simulink library "BEML_EMU_DoorsInput_Lib"  (R2019b)
settings: Solver=VariableStepAuto  StartTime=0.0  StopTime=10.0  RelTol=1e-3
undefined symbols (not defined in the file): DoorsSampleTime, DoorWinder, ElectricalSignals, EmerDoorLatched, EmerDoorOpenFault, EmergencyDoorGasSpring, EmergencyDoorHandle, EmergencyDoorMechanicalUnlocked, HasCab, InputControlStates, RampCoverLockingLever, RampHandle, RampMiddleSupport, RampWinder
libraries: simulink x128, $bdroot x8, VectorOperationsLib x1
(part 2 of 2)

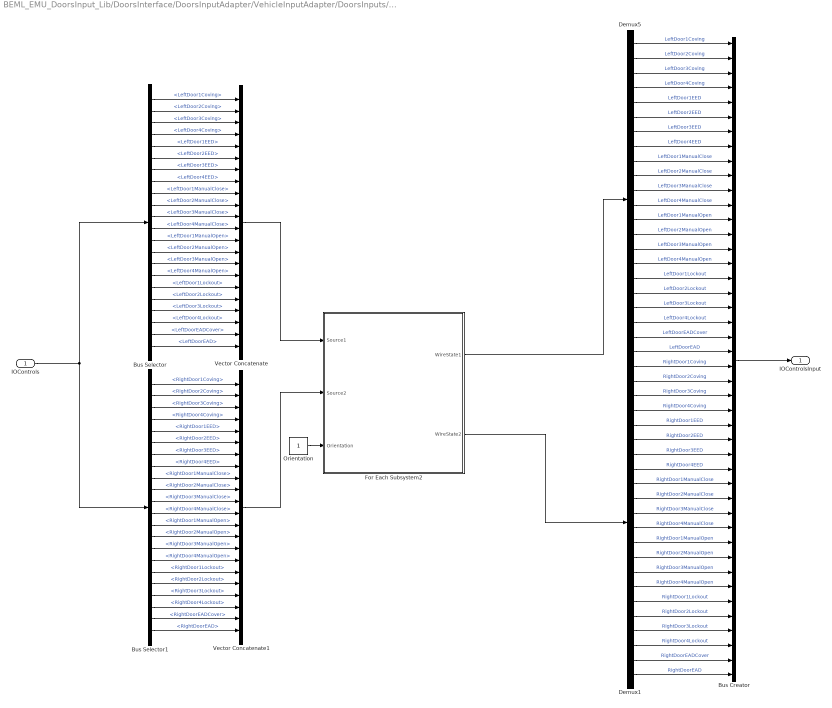
== system BEML_EMU_DoorsInput_Lib/DoorsInterface/DoorsInputAdapter/VehicleInputAdapter/DoorsInputs/DoorsArrangement/Subsystem1 ==
  IOControls : Inport
  Bus Creator : BusCreator  Inputs=LeftDoor1Coving,LeftDoor2Coving,LeftDoor3Coving,LeftDoor4Coving,LeftDoor1EED,LeftDoor2EED,LeftDoor3EED,LeftDoor4EED,LeftDoor1ManualClose,LeftDoor2ManualClose,LeftDoor3ManualClose,LeftDoor4ManualClose,LeftDoor1ManualOpen,LeftDoor2ManualOpen,LeftDoor3ManualOpen,LeftDoor4ManualOpen,LeftDoor1Lockout,LeftDoor2Lockout,LeftDoor3Lockout,LeftDoor4Lockout,LeftDoorEADCover,LeftDoorEAD,RightDoor1Coving,RightDoor2Coving,RightDoor3Coving,RightDoor4Coving,RightDoor1EED,RightDoor2EED,RightDoor3EED,RightDoor4EED,RightDoor1ManualClose,RightDoor2ManualClose,RightDoor3ManualClose,RightDoor4ManualClose,RightDoor1ManualOpen,RightDoor2ManualOpen,RightDoor3ManualOpen,RightDoor4ManualOpen,RightDoor1Lockout,RightDoor2Lockout,RightDoor3Lockout,RightDoor4Lockout,RightDoorEADCover,RightDoorEAD
  Bus Selector : BusSelector  OutputSignals=LeftDoor1Coving,LeftDoor2Coving,LeftDoor3Coving,LeftDoor4Coving,LeftDoor1EED,LeftDoor2EED,LeftDoor3EED,LeftDoor4EED,LeftDoor1ManualClose,LeftDoor2ManualClose,LeftDoor3ManualClose,LeftDoor4ManualClose,LeftDoor1ManualOpen,LeftDoor2ManualOpen,LeftDoor3ManualOpen,LeftDoor4ManualOpen,LeftDoor1Lockout,LeftDoor2Lockout,LeftDoor3Lockout,LeftDoor4Lockout,LeftDoorEADCover,LeftDoorEAD
  Bus Selector1 : BusSelector  OutputSignals=RightDoor1Coving,RightDoor2Coving,RightDoor3Coving,RightDoor4Coving,RightDoor1EED,RightDoor2EED,RightDoor3EED,RightDoor4EED,RightDoor1ManualClose,RightDoor2ManualClose,RightDoor3ManualClose,RightDoor4ManualClose,RightDoor1ManualOpen,RightDoor2ManualOpen,RightDoor3ManualOpen,RightDoor4ManualOpen,RightDoor1Lockout,RightDoor2Lockout,RightDoor3Lockout,RightDoor4Lockout,RightDoorEADCover,RightDoorEAD
  Demux1 : Demux  Outputs=22
  Demux5 : Demux  Outputs=22
  For Each Subsystem2 : Subsystem  TreatAsAtomicUnit=on
  Orientation : Constant
  Vector Concatenate : Concatenate  NumInputs=22
  Vector Concatenate1 : Concatenate  NumInputs=22
  IOControlsInput : Outport
  wires:
  Bus Selector/22 -> Vector Concatenate/22  "<LeftDoorEAD>"
  Bus Selector/21 -> Vector Concatenate/21  "<LeftDoorEADCover>"
  Bus Selector/1 -> Vector Concatenate/1  "<LeftDoor1Coving>"
  Bus Selector/2 -> Vector Concatenate/2  "<LeftDoor2Coving>"
  Bus Selector/3 -> Vector Concatenate/3  "<LeftDoor3Coving>"
  Bus Selector/4 -> Vector Concatenate/4  "<LeftDoor4Coving>"
  Bus Selector/5 -> Vector Concatenate/5  "<LeftDoor1EED>"
  Bus Selector/6 -> Vector Concatenate/6  "<LeftDoor2EED>"
  Bus Selector/7 -> Vector Concatenate/7  "<LeftDoor3EED>"
  Bus Selector/8 -> Vector Concatenate/8  "<LeftDoor4EED>"
  Bus Selector/9 -> Vector Concatenate/9  "<LeftDoor1ManualClose>"
  Bus Selector/10 -> Vector Concatenate/10  "<LeftDoor2ManualClose>"
  Bus Selector/11 -> Vector Concatenate/11  "<LeftDoor3ManualClose>"
  Bus Selector/12 -> Vector Concatenate/12  "<LeftDoor4ManualClose>"
  Bus Selector/13 -> Vector Concatenate/13  "<LeftDoor1ManualOpen>"
  Bus Selector/14 -> Vector Concatenate/14  "<LeftDoor2ManualOpen>"
  Bus Selector/15 -> Vector Concatenate/15  "<LeftDoor3ManualOpen>"
  Bus Selector/16 -> Vector Concatenate/16  "<LeftDoor4ManualOpen>"
  Bus Selector/17 -> Vector Concatenate/17  "<LeftDoor1Lockout>"
  Bus Selector/18 -> Vector Concatenate/18  "<LeftDoor2Lockout>"
  Bus Selector/19 -> Vector Concatenate/19  "<LeftDoor3Lockout>"
  Bus Selector/20 -> Vector Concatenate/20  "<LeftDoor4Lockout>"
  Bus Selector1/20 -> Vector Concatenate1/20  "<RightDoor4Lockout>"
  Bus Selector1/19 -> Vector Concatenate1/19  "<RightDoor3Lockout>"
  Bus Selector1/18 -> Vector Concatenate1/18  "<RightDoor2Lockout>"
  Bus Selector1/17 -> Vector Concatenate1/17  "<RightDoor1Lockout>"
  Bus Selector1/16 -> Vector Concatenate1/16  "<RightDoor4ManualOpen>"
  Bus Selector1/15 -> Vector Concatenate1/15  "<RightDoor3ManualOpen>"
  Bus Selector1/14 -> Vector Concatenate1/14  "<RightDoor2ManualOpen>"
  Bus Selector1/13 -> Vector Concatenate1/13  "<RightDoor1ManualOpen>"
  Bus Selector1/12 -> Vector Concatenate1/12  "<RightDoor4ManualClose>"
  Bus Selector1/11 -> Vector Concatenate1/11  "<RightDoor3ManualClose>"
  Bus Selector1/10 -> Vector Concatenate1/10  "<RightDoor2ManualClose>"
  Bus Selector1/9 -> Vector Concatenate1/9  "<RightDoor1ManualClose>"
  Bus Selector1/8 -> Vector Concatenate1/8  "<RightDoor4EED>"
  Bus Selector1/7 -> Vector Concatenate1/7  "<RightDoor3EED>"
  Bus Selector1/6 -> Vector Concatenate1/6  "<RightDoor2EED>"
  Bus Selector1/5 -> Vector Concatenate1/5  "<RightDoor1EED>"
  Bus Selector1/4 -> Vector Concatenate1/4  "<RightDoor4Coving>"
  Bus Selector1/3 -> Vector Concatenate1/3  "<RightDoor3Coving>"
  Bus Selector1/2 -> Vector Concatenate1/2  "<RightDoor2Coving>"
  Bus Selector1/1 -> Vector Concatenate1/1  "<RightDoor1Coving>"
  Bus Selector1/21 -> Vector Concatenate1/21  "<RightDoorEADCover>"
  Bus Selector1/22 -> Vector Concatenate1/22  "<RightDoorEAD>"
  IOControls/1 -> Bus Selector/1, Bus Selector1/1
  Vector Concatenate/1 -> For Each Subsystem2/1(Source1)
  Vector Concatenate1/1 -> For Each Subsystem2/2(Source2)
  For Each Subsystem2/2(WireState2) -> Demux1/1
  For Each Subsystem2/1(WireState1) -> Demux5/1
  Demux5/22 -> Bus Creator/22  "LeftDoorEAD"
  Demux5/21 -> Bus Creator/21  "LeftDoorEADCover"
  Demux5/20 -> Bus Creator/20  "LeftDoor4Lockout"
  Demux5/19 -> Bus Creator/19  "LeftDoor3Lockout"
  Demux5/18 -> Bus Creator/18  "LeftDoor2Lockout"
  Demux5/17 -> Bus Creator/17  "LeftDoor1Lockout"
  Demux5/16 -> Bus Creator/16  "LeftDoor4ManualOpen"
  Demux5/15 -> Bus Creator/15  "LeftDoor3ManualOpen"
  Demux5/14 -> Bus Creator/14  "LeftDoor2ManualOpen"
  Demux5/13 -> Bus Creator/13  "LeftDoor1ManualOpen"
  Demux5/12 -> Bus Creator/12  "LeftDoor4ManualClose"
  Demux5/11 -> Bus Creator/11  "LeftDoor3ManualClose"
  Demux5/10 -> Bus Creator/10  "LeftDoor2ManualClose"
  Demux5/9 -> Bus Creator/9  "LeftDoor1ManualClose"
  Demux5/8 -> Bus Creator/8  "LeftDoor4EED"
  Demux5/7 -> Bus Creator/7  "LeftDoor3EED"
  Demux5/6 -> Bus Creator/6  "LeftDoor2EED"
  Demux5/5 -> Bus Creator/5  "LeftDoor1EED"
  Demux5/4 -> Bus Creator/4  "LeftDoor4Coving"
  Demux5/3 -> Bus Creator/3  "LeftDoor3Coving"
  Demux5/2 -> Bus Creator/2  "LeftDoor2Coving"
  Demux5/1 -> Bus Creator/1  "LeftDoor1Coving"
  Demux1/1 -> Bus Creator/23  "RightDoor1Coving"
  Demux1/2 -> Bus Creator/24  "RightDoor2Coving"
  Demux1/3 -> Bus Creator/25  "RightDoor3Coving"
  Demux1/4 -> Bus Creator/26  "RightDoor4Coving"
  Demux1/5 -> Bus Creator/27  "RightDoor1EED"
  Demux1/6 -> Bus Creator/28  "RightDoor2EED"
  Demux1/7 -> Bus Creator/29  "RightDoor3EED"
  Demux1/8 -> Bus Creator/30  "RightDoor4EED"
  Demux1/9 -> Bus Creator/31  "RightDoor1ManualClose"
  Demux1/10 -> Bus Creator/32  "RightDoor2ManualClose"
  Demux1/11 -> Bus Creator/33  "RightDoor3ManualClose"
  Demux1/12 -> Bus Creator/34  "RightDoor4ManualClose"
  Demux1/13 -> Bus Creator/35  "RightDoor1ManualOpen"
  Demux1/14 -> Bus Creator/36  "RightDoor2ManualOpen"
  Demux1/15 -> Bus Creator/37  "RightDoor3ManualOpen"
  Demux1/16 -> Bus Creator/38  "RightDoor4ManualOpen"
  Demux1/17 -> Bus Creator/39  "RightDoor1Lockout"
  Demux1/18 -> Bus Creator/40  "RightDoor2Lockout"
  Demux1/19 -> Bus Creator/41  "RightDoor3Lockout"
  Demux1/20 -> Bus Creator/42  "RightDoor4Lockout"
  Demux1/21 -> Bus Creator/43  "RightDoorEADCover"
  Demux1/22 -> Bus Creator/44  "RightDoorEAD"
  Bus Creator/1 -> IOControlsInput/1
  Orientation/1 -> For Each Subsystem2/3(Orientation)

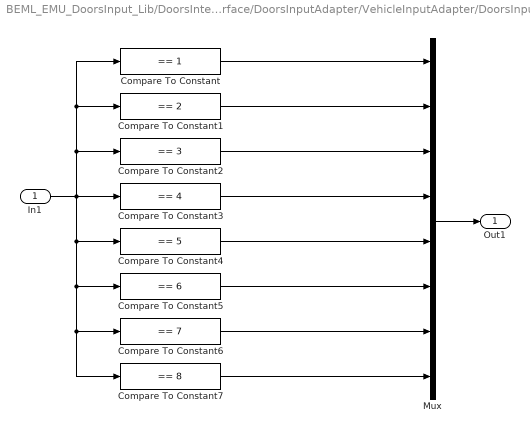
== system BEML_EMU_DoorsInput_Lib/DoorsInterface/DoorsInputAdapter/VehicleInputAdapter/DoorsInputs/Subsystem/Subsystem ==
  In1 : Inport
  Compare To Constant : simulink/Logic and Bit Operations/Compare To Constant  relop===  const=1  OutDataTypeStr=boolean
  Compare To Constant1 : simulink/Logic and Bit Operations/Compare To Constant  relop===  const=2  OutDataTypeStr=boolean
  Compare To Constant2 : simulink/Logic and Bit Operations/Compare To Constant  relop===  const=3  OutDataTypeStr=boolean
  Compare To Constant3 : simulink/Logic and Bit Operations/Compare To Constant  relop===  const=4  OutDataTypeStr=boolean
  Compare To Constant4 : simulink/Logic and Bit Operations/Compare To Constant  relop===  const=5  OutDataTypeStr=boolean
  Compare To Constant5 : simulink/Logic and Bit Operations/Compare To Constant  relop===  const=6  OutDataTypeStr=boolean
  Compare To Constant6 : simulink/Logic and Bit Operations/Compare To Constant  relop===  const=7  OutDataTypeStr=boolean
  Compare To Constant7 : simulink/Logic and Bit Operations/Compare To Constant  relop===  const=8  OutDataTypeStr=boolean
  Mux : Mux  Inputs=8
  Out1 : Outport
  wires:
  Compare To Constant7/1 -> Mux/8
  Compare To Constant6/1 -> Mux/7
  Compare To Constant5/1 -> Mux/6
  Compare To Constant4/1 -> Mux/5
  Compare To Constant3/1 -> Mux/4
  Compare To Constant2/1 -> Mux/3
  Compare To Constant1/1 -> Mux/2
  Compare To Constant/1 -> Mux/1
  Mux/1 -> Out1/1
  In1/1 -> Compare To Constant4/1, Compare To Constant5/1, Compare To Constant6/1, Compare To Constant7/1, Compare To Constant3/1, Compare To Constant2/1, Compare To Constant1/1, Compare To Constant/1

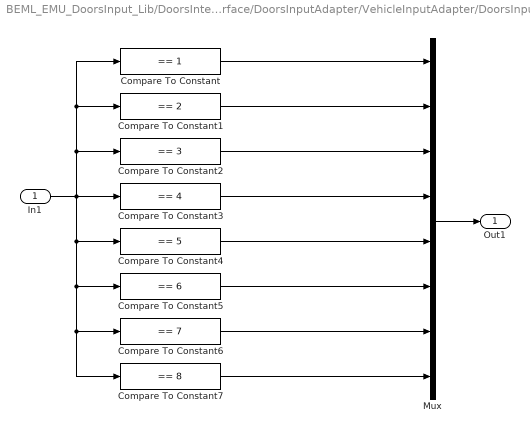
== system BEML_EMU_DoorsInput_Lib/DoorsInterface/DoorsInputAdapter/VehicleInputAdapter/DoorsInputs/Subsystem/Subsystem1 ==
  In1 : Inport
  Compare To Constant : simulink/Logic and Bit Operations/Compare To Constant  relop===  const=1  OutDataTypeStr=boolean
  Compare To Constant1 : simulink/Logic and Bit Operations/Compare To Constant  relop===  const=2  OutDataTypeStr=boolean
  Compare To Constant2 : simulink/Logic and Bit Operations/Compare To Constant  relop===  const=3  OutDataTypeStr=boolean
  Compare To Constant3 : simulink/Logic and Bit Operations/Compare To Constant  relop===  const=4  OutDataTypeStr=boolean
  Compare To Constant4 : simulink/Logic and Bit Operations/Compare To Constant  relop===  const=5  OutDataTypeStr=boolean
  Compare To Constant5 : simulink/Logic and Bit Operations/Compare To Constant  relop===  const=6  OutDataTypeStr=boolean
  Compare To Constant6 : simulink/Logic and Bit Operations/Compare To Constant  relop===  const=7  OutDataTypeStr=boolean
  Compare To Constant7 : simulink/Logic and Bit Operations/Compare To Constant  relop===  const=8  OutDataTypeStr=boolean
  Mux : Mux  Inputs=8
  Out1 : Outport
  wires:
  In1/1 -> Compare To Constant/1, Compare To Constant1/1, Compare To Constant2/1, Compare To Constant3/1, Compare To Constant7/1, Compare To Constant6/1, Compare To Constant5/1, Compare To Constant4/1
  Mux/1 -> Out1/1
  Compare To Constant/1 -> Mux/1
  Compare To Constant1/1 -> Mux/2
  Compare To Constant2/1 -> Mux/3
  Compare To Constant3/1 -> Mux/4
  Compare To Constant4/1 -> Mux/5
  Compare To Constant5/1 -> Mux/6
  Compare To Constant6/1 -> Mux/7
  Compare To Constant7/1 -> Mux/8

== system BEML_EMU_DoorsInput_Lib/DoorsInterface/DoorsInputAdapter/VehicleInputAdapter/DoorsInputs/Subsystem/Subsystem10 ==
  In1 : Inport
  Compare To Constant : simulink/Logic and Bit Operations/Compare To Constant  relop===  const=1  OutDataTypeStr=boolean
  Compare To Constant1 : simulink/Logic and Bit Operations/Compare To Constant  relop===  const=2  OutDataTypeStr=boolean
  Compare To Constant2 : simulink/Logic and Bit Operations/Compare To Constant  relop===  const=3  OutDataTypeStr=boolean
  Compare To Constant3 : simulink/Logic and Bit Operations/Compare To Constant  relop===  const=4  OutDataTypeStr=boolean
  Compare To Constant4 : simulink/Logic and Bit Operations/Compare To Constant  relop===  const=5  OutDataTypeStr=boolean
  Compare To Constant5 : simulink/Logic and Bit Operations/Compare To Constant  relop===  const=6  OutDataTypeStr=boolean
  Compare To Constant6 : simulink/Logic and Bit Operations/Compare To Constant  relop===  const=7  OutDataTypeStr=boolean
  Compare To Constant7 : simulink/Logic and Bit Operations/Compare To Constant  relop===  const=8  OutDataTypeStr=boolean
  Mux : Mux  Inputs=8
  Out1 : Outport
  wires:
  Compare To Constant7/1 -> Mux/8
  Compare To Constant6/1 -> Mux/7
  Compare To Constant5/1 -> Mux/6
  Compare To Constant4/1 -> Mux/5
  Compare To Constant3/1 -> Mux/4
  Compare To Constant2/1 -> Mux/3
  Compare To Constant1/1 -> Mux/2
  Compare To Constant/1 -> Mux/1
  Mux/1 -> Out1/1
  In1/1 -> Compare To Constant4/1, Compare To Constant5/1, Compare To Constant6/1, Compare To Constant7/1, Compare To Constant3/1, Compare To Constant2/1, Compare To Constant1/1, Compare To Constant/1

== system BEML_EMU_DoorsInput_Lib/DoorsInterface/DoorsInputAdapter/VehicleInputAdapter/DoorsInputs/Subsystem/Subsystem11 ==
  In1 : Inport
  Compare To Constant : simulink/Logic and Bit Operations/Compare To Constant  relop===  const=1  OutDataTypeStr=boolean
  Compare To Constant1 : simulink/Logic and Bit Operations/Compare To Constant  relop===  const=2  OutDataTypeStr=boolean
  Compare To Constant2 : simulink/Logic and Bit Operations/Compare To Constant  relop===  const=3  OutDataTypeStr=boolean
  Compare To Constant3 : simulink/Logic and Bit Operations/Compare To Constant  relop===  const=4  OutDataTypeStr=boolean
  Compare To Constant4 : simulink/Logic and Bit Operations/Compare To Constant  relop===  const=5  OutDataTypeStr=boolean
  Compare To Constant5 : simulink/Logic and Bit Operations/Compare To Constant  relop===  const=6  OutDataTypeStr=boolean
  Compare To Constant6 : simulink/Logic and Bit Operations/Compare To Constant  relop===  const=7  OutDataTypeStr=boolean
  Compare To Constant7 : simulink/Logic and Bit Operations/Compare To Constant  relop===  const=8  OutDataTypeStr=boolean
  Mux : Mux  Inputs=8
  Out1 : Outport
  wires:
  In1/1 -> Compare To Constant/1, Compare To Constant1/1, Compare To Constant2/1, Compare To Constant3/1, Compare To Constant7/1, Compare To Constant6/1, Compare To Constant5/1, Compare To Constant4/1
  Mux/1 -> Out1/1
  Compare To Constant/1 -> Mux/1
  Compare To Constant1/1 -> Mux/2
  Compare To Constant2/1 -> Mux/3
  Compare To Constant3/1 -> Mux/4
  Compare To Constant4/1 -> Mux/5
  Compare To Constant5/1 -> Mux/6
  Compare To Constant6/1 -> Mux/7
  Compare To Constant7/1 -> Mux/8

== system BEML_EMU_DoorsInput_Lib/DoorsInterface/DoorsInputAdapter/VehicleInputAdapter/DoorsInputs/Subsystem/Subsystem12 ==
  In1 : Inport
  Compare To Constant : simulink/Logic and Bit Operations/Compare To Constant  relop===  const=1  OutDataTypeStr=boolean
  Compare To Constant1 : simulink/Logic and Bit Operations/Compare To Constant  relop===  const=2  OutDataTypeStr=boolean
  Compare To Constant2 : simulink/Logic and Bit Operations/Compare To Constant  relop===  const=3  OutDataTypeStr=boolean
  Compare To Constant3 : simulink/Logic and Bit Operations/Compare To Constant  relop===  const=4  OutDataTypeStr=boolean
  Compare To Constant4 : simulink/Logic and Bit Operations/Compare To Constant  relop===  const=5  OutDataTypeStr=boolean
  Compare To Constant5 : simulink/Logic and Bit Operations/Compare To Constant  relop===  const=6  OutDataTypeStr=boolean
  Compare To Constant6 : simulink/Logic and Bit Operations/Compare To Constant  relop===  const=7  OutDataTypeStr=boolean
  Compare To Constant7 : simulink/Logic and Bit Operations/Compare To Constant  relop===  const=8  OutDataTypeStr=boolean
  Mux : Mux  Inputs=8
  Out1 : Outport
  wires:
  Compare To Constant7/1 -> Mux/8
  Compare To Constant6/1 -> Mux/7
  Compare To Constant5/1 -> Mux/6
  Compare To Constant4/1 -> Mux/5
  Compare To Constant3/1 -> Mux/4
  Compare To Constant2/1 -> Mux/3
  Compare To Constant1/1 -> Mux/2
  Compare To Constant/1 -> Mux/1
  Mux/1 -> Out1/1
  In1/1 -> Compare To Constant4/1, Compare To Constant5/1, Compare To Constant6/1, Compare To Constant7/1, Compare To Constant3/1, Compare To Constant2/1, Compare To Constant1/1, Compare To Constant/1

== system BEML_EMU_DoorsInput_Lib/DoorsInterface/DoorsInputAdapter/VehicleInputAdapter/DoorsInputs/Subsystem/Subsystem13 ==
  In1 : Inport
  Compare To Constant : simulink/Logic and Bit Operations/Compare To Constant  relop===  const=1  OutDataTypeStr=boolean
  Compare To Constant1 : simulink/Logic and Bit Operations/Compare To Constant  relop===  const=2  OutDataTypeStr=boolean
  Compare To Constant2 : simulink/Logic and Bit Operations/Compare To Constant  relop===  const=3  OutDataTypeStr=boolean
  Compare To Constant3 : simulink/Logic and Bit Operations/Compare To Constant  relop===  const=4  OutDataTypeStr=boolean
  Compare To Constant4 : simulink/Logic and Bit Operations/Compare To Constant  relop===  const=5  OutDataTypeStr=boolean
  Compare To Constant5 : simulink/Logic and Bit Operations/Compare To Constant  relop===  const=6  OutDataTypeStr=boolean
  Compare To Constant6 : simulink/Logic and Bit Operations/Compare To Constant  relop===  const=7  OutDataTypeStr=boolean
  Compare To Constant7 : simulink/Logic and Bit Operations/Compare To Constant  relop===  const=8  OutDataTypeStr=boolean
  Mux : Mux  Inputs=8
  Out1 : Outport
  wires:
  In1/1 -> Compare To Constant/1, Compare To Constant1/1, Compare To Constant2/1, Compare To Constant3/1, Compare To Constant7/1, Compare To Constant6/1, Compare To Constant5/1, Compare To Constant4/1
  Mux/1 -> Out1/1
  Compare To Constant/1 -> Mux/1
  Compare To Constant1/1 -> Mux/2
  Compare To Constant2/1 -> Mux/3
  Compare To Constant3/1 -> Mux/4
  Compare To Constant4/1 -> Mux/5
  Compare To Constant5/1 -> Mux/6
  Compare To Constant6/1 -> Mux/7
  Compare To Constant7/1 -> Mux/8

== system BEML_EMU_DoorsInput_Lib/DoorsInterface/DoorsInputAdapter/VehicleInputAdapter/DoorsInputs/Subsystem/Subsystem14 ==
  In1 : Inport
  Compare To Constant : simulink/Logic and Bit Operations/Compare To Constant  relop===  const=1  OutDataTypeStr=boolean
  Compare To Constant1 : simulink/Logic and Bit Operations/Compare To Constant  relop===  const=2  OutDataTypeStr=boolean
  Compare To Constant2 : simulink/Logic and Bit Operations/Compare To Constant  relop===  const=3  OutDataTypeStr=boolean
  Compare To Constant3 : simulink/Logic and Bit Operations/Compare To Constant  relop===  const=4  OutDataTypeStr=boolean
  Compare To Constant4 : simulink/Logic and Bit Operations/Compare To Constant  relop===  const=5  OutDataTypeStr=boolean
  Compare To Constant5 : simulink/Logic and Bit Operations/Compare To Constant  relop===  const=6  OutDataTypeStr=boolean
  Compare To Constant6 : simulink/Logic and Bit Operations/Compare To Constant  relop===  const=7  OutDataTypeStr=boolean
  Compare To Constant7 : simulink/Logic and Bit Operations/Compare To Constant  relop===  const=8  OutDataTypeStr=boolean
  Mux : Mux  Inputs=8
  Out1 : Outport
  wires:
  Compare To Constant7/1 -> Mux/8
  Compare To Constant6/1 -> Mux/7
  Compare To Constant5/1 -> Mux/6
  Compare To Constant4/1 -> Mux/5
  Compare To Constant3/1 -> Mux/4
  Compare To Constant2/1 -> Mux/3
  Compare To Constant1/1 -> Mux/2
  Compare To Constant/1 -> Mux/1
  Mux/1 -> Out1/1
  In1/1 -> Compare To Constant4/1, Compare To Constant5/1, Compare To Constant6/1, Compare To Constant7/1, Compare To Constant3/1, Compare To Constant2/1, Compare To Constant1/1, Compare To Constant/1

== system BEML_EMU_DoorsInput_Lib/DoorsInterface/DoorsInputAdapter/VehicleInputAdapter/DoorsInputs/Subsystem/Subsystem15 ==
  In1 : Inport
  Compare To Constant : simulink/Logic and Bit Operations/Compare To Constant  relop===  const=1  OutDataTypeStr=boolean
  Compare To Constant1 : simulink/Logic and Bit Operations/Compare To Constant  relop===  const=2  OutDataTypeStr=boolean
  Compare To Constant2 : simulink/Logic and Bit Operations/Compare To Constant  relop===  const=3  OutDataTypeStr=boolean
  Compare To Constant3 : simulink/Logic and Bit Operations/Compare To Constant  relop===  const=4  OutDataTypeStr=boolean
  Compare To Constant4 : simulink/Logic and Bit Operations/Compare To Constant  relop===  const=5  OutDataTypeStr=boolean
  Compare To Constant5 : simulink/Logic and Bit Operations/Compare To Constant  relop===  const=6  OutDataTypeStr=boolean
  Compare To Constant6 : simulink/Logic and Bit Operations/Compare To Constant  relop===  const=7  OutDataTypeStr=boolean
  Compare To Constant7 : simulink/Logic and Bit Operations/Compare To Constant  relop===  const=8  OutDataTypeStr=boolean
  Mux : Mux  Inputs=8
  Out1 : Outport
  wires:
  In1/1 -> Compare To Constant/1, Compare To Constant1/1, Compare To Constant2/1, Compare To Constant3/1, Compare To Constant7/1, Compare To Constant6/1, Compare To Constant5/1, Compare To Constant4/1
  Mux/1 -> Out1/1
  Compare To Constant/1 -> Mux/1
  Compare To Constant1/1 -> Mux/2
  Compare To Constant2/1 -> Mux/3
  Compare To Constant3/1 -> Mux/4
  Compare To Constant4/1 -> Mux/5
  Compare To Constant5/1 -> Mux/6
  Compare To Constant6/1 -> Mux/7
  Compare To Constant7/1 -> Mux/8

== system BEML_EMU_DoorsInput_Lib/DoorsInterface/DoorsInputAdapter/VehicleInputAdapter/DoorsInputs/Subsystem/Subsystem2 ==
  In1 : Inport
  Compare To Constant : simulink/Logic and Bit Operations/Compare To Constant  relop===  const=1  OutDataTypeStr=boolean
  Compare To Constant1 : simulink/Logic and Bit Operations/Compare To Constant  relop===  const=2  OutDataTypeStr=boolean
  Compare To Constant2 : simulink/Logic and Bit Operations/Compare To Constant  relop===  const=3  OutDataTypeStr=boolean
  Compare To Constant3 : simulink/Logic and Bit Operations/Compare To Constant  relop===  const=4  OutDataTypeStr=boolean
  Compare To Constant4 : simulink/Logic and Bit Operations/Compare To Constant  relop===  const=5  OutDataTypeStr=boolean
  Compare To Constant5 : simulink/Logic and Bit Operations/Compare To Constant  relop===  const=6  OutDataTypeStr=boolean
  Compare To Constant6 : simulink/Logic and Bit Operations/Compare To Constant  relop===  const=7  OutDataTypeStr=boolean
  Compare To Constant7 : simulink/Logic and Bit Operations/Compare To Constant  relop===  const=8  OutDataTypeStr=boolean
  Mux : Mux  Inputs=8
  Out1 : Outport
  wires:
  Compare To Constant7/1 -> Mux/8
  Compare To Constant6/1 -> Mux/7
  Compare To Constant5/1 -> Mux/6
  Compare To Constant4/1 -> Mux/5
  Compare To Constant3/1 -> Mux/4
  Compare To Constant2/1 -> Mux/3
  Compare To Constant1/1 -> Mux/2
  Compare To Constant/1 -> Mux/1
  Mux/1 -> Out1/1
  In1/1 -> Compare To Constant4/1, Compare To Constant5/1, Compare To Constant6/1, Compare To Constant7/1, Compare To Constant3/1, Compare To Constant2/1, Compare To Constant1/1, Compare To Constant/1

== system BEML_EMU_DoorsInput_Lib/DoorsInterface/DoorsInputAdapter/VehicleInputAdapter/DoorsInputs/Subsystem/Subsystem3 ==
  In1 : Inport
  Compare To Constant : simulink/Logic and Bit Operations/Compare To Constant  relop===  const=1  OutDataTypeStr=boolean
  Compare To Constant1 : simulink/Logic and Bit Operations/Compare To Constant  relop===  const=2  OutDataTypeStr=boolean
  Compare To Constant2 : simulink/Logic and Bit Operations/Compare To Constant  relop===  const=3  OutDataTypeStr=boolean
  Compare To Constant3 : simulink/Logic and Bit Operations/Compare To Constant  relop===  const=4  OutDataTypeStr=boolean
  Compare To Constant4 : simulink/Logic and Bit Operations/Compare To Constant  relop===  const=5  OutDataTypeStr=boolean
  Compare To Constant5 : simulink/Logic and Bit Operations/Compare To Constant  relop===  const=6  OutDataTypeStr=boolean
  Compare To Constant6 : simulink/Logic and Bit Operations/Compare To Constant  relop===  const=7  OutDataTypeStr=boolean
  Compare To Constant7 : simulink/Logic and Bit Operations/Compare To Constant  relop===  const=8  OutDataTypeStr=boolean
  Mux : Mux  Inputs=8
  Out1 : Outport
  wires:
  In1/1 -> Compare To Constant/1, Compare To Constant1/1, Compare To Constant2/1, Compare To Constant3/1, Compare To Constant7/1, Compare To Constant6/1, Compare To Constant5/1, Compare To Constant4/1
  Mux/1 -> Out1/1
  Compare To Constant/1 -> Mux/1
  Compare To Constant1/1 -> Mux/2
  Compare To Constant2/1 -> Mux/3
  Compare To Constant3/1 -> Mux/4
  Compare To Constant4/1 -> Mux/5
  Compare To Constant5/1 -> Mux/6
  Compare To Constant6/1 -> Mux/7
  Compare To Constant7/1 -> Mux/8

== system BEML_EMU_DoorsInput_Lib/DoorsInterface/DoorsInputAdapter/VehicleInputAdapter/DoorsInputs/Subsystem/Subsystem4 ==
  In1 : Inport
  Compare To Constant : simulink/Logic and Bit Operations/Compare To Constant  relop===  const=1  OutDataTypeStr=boolean
  Compare To Constant1 : simulink/Logic and Bit Operations/Compare To Constant  relop===  const=2  OutDataTypeStr=boolean
  Compare To Constant2 : simulink/Logic and Bit Operations/Compare To Constant  relop===  const=3  OutDataTypeStr=boolean
  Compare To Constant3 : simulink/Logic and Bit Operations/Compare To Constant  relop===  const=4  OutDataTypeStr=boolean
  Compare To Constant4 : simulink/Logic and Bit Operations/Compare To Constant  relop===  const=5  OutDataTypeStr=boolean
  Compare To Constant5 : simulink/Logic and Bit Operations/Compare To Constant  relop===  const=6  OutDataTypeStr=boolean
  Compare To Constant6 : simulink/Logic and Bit Operations/Compare To Constant  relop===  const=7  OutDataTypeStr=boolean
  Compare To Constant7 : simulink/Logic and Bit Operations/Compare To Constant  relop===  const=8  OutDataTypeStr=boolean
  Mux : Mux  Inputs=8
  Out1 : Outport
  wires:
  Compare To Constant7/1 -> Mux/8
  Compare To Constant6/1 -> Mux/7
  Compare To Constant5/1 -> Mux/6
  Compare To Constant4/1 -> Mux/5
  Compare To Constant3/1 -> Mux/4
  Compare To Constant2/1 -> Mux/3
  Compare To Constant1/1 -> Mux/2
  Compare To Constant/1 -> Mux/1
  Mux/1 -> Out1/1
  In1/1 -> Compare To Constant4/1, Compare To Constant5/1, Compare To Constant6/1, Compare To Constant7/1, Compare To Constant3/1, Compare To Constant2/1, Compare To Constant1/1, Compare To Constant/1

== system BEML_EMU_DoorsInput_Lib/DoorsInterface/DoorsInputAdapter/VehicleInputAdapter/DoorsInputs/Subsystem/Subsystem5 ==
  In1 : Inport
  Compare To Constant : simulink/Logic and Bit Operations/Compare To Constant  relop===  const=1  OutDataTypeStr=boolean
  Compare To Constant1 : simulink/Logic and Bit Operations/Compare To Constant  relop===  const=2  OutDataTypeStr=boolean
  Compare To Constant2 : simulink/Logic and Bit Operations/Compare To Constant  relop===  const=3  OutDataTypeStr=boolean
  Compare To Constant3 : simulink/Logic and Bit Operations/Compare To Constant  relop===  const=4  OutDataTypeStr=boolean
  Compare To Constant4 : simulink/Logic and Bit Operations/Compare To Constant  relop===  const=5  OutDataTypeStr=boolean
  Compare To Constant5 : simulink/Logic and Bit Operations/Compare To Constant  relop===  const=6  OutDataTypeStr=boolean
  Compare To Constant6 : simulink/Logic and Bit Operations/Compare To Constant  relop===  const=7  OutDataTypeStr=boolean
  Compare To Constant7 : simulink/Logic and Bit Operations/Compare To Constant  relop===  const=8  OutDataTypeStr=boolean
  Mux : Mux  Inputs=8
  Out1 : Outport
  wires:
  In1/1 -> Compare To Constant/1, Compare To Constant1/1, Compare To Constant2/1, Compare To Constant3/1, Compare To Constant7/1, Compare To Constant6/1, Compare To Constant5/1, Compare To Constant4/1
  Mux/1 -> Out1/1
  Compare To Constant/1 -> Mux/1
  Compare To Constant1/1 -> Mux/2
  Compare To Constant2/1 -> Mux/3
  Compare To Constant3/1 -> Mux/4
  Compare To Constant4/1 -> Mux/5
  Compare To Constant5/1 -> Mux/6
  Compare To Constant6/1 -> Mux/7
  Compare To Constant7/1 -> Mux/8

== system BEML_EMU_DoorsInput_Lib/DoorsInterface/DoorsInputAdapter/VehicleInputAdapter/DoorsInputs/Subsystem/Subsystem6 ==
  In1 : Inport
  Compare To Constant : simulink/Logic and Bit Operations/Compare To Constant  relop===  const=1  OutDataTypeStr=boolean
  Compare To Constant1 : simulink/Logic and Bit Operations/Compare To Constant  relop===  const=2  OutDataTypeStr=boolean
  Compare To Constant2 : simulink/Logic and Bit Operations/Compare To Constant  relop===  const=3  OutDataTypeStr=boolean
  Compare To Constant3 : simulink/Logic and Bit Operations/Compare To Constant  relop===  const=4  OutDataTypeStr=boolean
  Compare To Constant4 : simulink/Logic and Bit Operations/Compare To Constant  relop===  const=5  OutDataTypeStr=boolean
  Compare To Constant5 : simulink/Logic and Bit Operations/Compare To Constant  relop===  const=6  OutDataTypeStr=boolean
  Compare To Constant6 : simulink/Logic and Bit Operations/Compare To Constant  relop===  const=7  OutDataTypeStr=boolean
  Compare To Constant7 : simulink/Logic and Bit Operations/Compare To Constant  relop===  const=8  OutDataTypeStr=boolean
  Mux : Mux  Inputs=8
  Out1 : Outport
  wires:
  Compare To Constant7/1 -> Mux/8
  Compare To Constant6/1 -> Mux/7
  Compare To Constant5/1 -> Mux/6
  Compare To Constant4/1 -> Mux/5
  Compare To Constant3/1 -> Mux/4
  Compare To Constant2/1 -> Mux/3
  Compare To Constant1/1 -> Mux/2
  Compare To Constant/1 -> Mux/1
  Mux/1 -> Out1/1
  In1/1 -> Compare To Constant4/1, Compare To Constant5/1, Compare To Constant6/1, Compare To Constant7/1, Compare To Constant3/1, Compare To Constant2/1, Compare To Constant1/1, Compare To Constant/1

== system BEML_EMU_DoorsInput_Lib/DoorsInterface/DoorsInputAdapter/VehicleInputAdapter/DoorsInputs/Subsystem/Subsystem7 ==
  In1 : Inport
  Compare To Constant : simulink/Logic and Bit Operations/Compare To Constant  relop===  const=1  OutDataTypeStr=boolean
  Compare To Constant1 : simulink/Logic and Bit Operations/Compare To Constant  relop===  const=2  OutDataTypeStr=boolean
  Compare To Constant2 : simulink/Logic and Bit Operations/Compare To Constant  relop===  const=3  OutDataTypeStr=boolean
  Compare To Constant3 : simulink/Logic and Bit Operations/Compare To Constant  relop===  const=4  OutDataTypeStr=boolean
  Compare To Constant4 : simulink/Logic and Bit Operations/Compare To Constant  relop===  const=5  OutDataTypeStr=boolean
  Compare To Constant5 : simulink/Logic and Bit Operations/Compare To Constant  relop===  const=6  OutDataTypeStr=boolean
  Compare To Constant6 : simulink/Logic and Bit Operations/Compare To Constant  relop===  const=7  OutDataTypeStr=boolean
  Compare To Constant7 : simulink/Logic and Bit Operations/Compare To Constant  relop===  const=8  OutDataTypeStr=boolean
  Mux : Mux  Inputs=8
  Out1 : Outport
  wires:
  In1/1 -> Compare To Constant/1, Compare To Constant1/1, Compare To Constant2/1, Compare To Constant3/1, Compare To Constant7/1, Compare To Constant6/1, Compare To Constant5/1, Compare To Constant4/1
  Mux/1 -> Out1/1
  Compare To Constant/1 -> Mux/1
  Compare To Constant1/1 -> Mux/2
  Compare To Constant2/1 -> Mux/3
  Compare To Constant3/1 -> Mux/4
  Compare To Constant4/1 -> Mux/5
  Compare To Constant5/1 -> Mux/6
  Compare To Constant6/1 -> Mux/7
  Compare To Constant7/1 -> Mux/8

== system BEML_EMU_DoorsInput_Lib/DoorsInterface/DoorsInputAdapter/VehicleInputAdapter/DoorsInputs/Subsystem/Subsystem8 ==
  In1 : Inport
  Compare To Constant : simulink/Logic and Bit Operations/Compare To Constant  relop===  const=1  OutDataTypeStr=boolean
  Compare To Constant1 : simulink/Logic and Bit Operations/Compare To Constant  relop===  const=2  OutDataTypeStr=boolean
  Compare To Constant2 : simulink/Logic and Bit Operations/Compare To Constant  relop===  const=3  OutDataTypeStr=boolean
  Compare To Constant3 : simulink/Logic and Bit Operations/Compare To Constant  relop===  const=4  OutDataTypeStr=boolean
  Compare To Constant4 : simulink/Logic and Bit Operations/Compare To Constant  relop===  const=5  OutDataTypeStr=boolean
  Compare To Constant5 : simulink/Logic and Bit Operations/Compare To Constant  relop===  const=6  OutDataTypeStr=boolean
  Compare To Constant6 : simulink/Logic and Bit Operations/Compare To Constant  relop===  const=7  OutDataTypeStr=boolean
  Compare To Constant7 : simulink/Logic and Bit Operations/Compare To Constant  relop===  const=8  OutDataTypeStr=boolean
  Mux : Mux  Inputs=8
  Out1 : Outport
  wires:
  Compare To Constant7/1 -> Mux/8
  Compare To Constant6/1 -> Mux/7
  Compare To Constant5/1 -> Mux/6
  Compare To Constant4/1 -> Mux/5
  Compare To Constant3/1 -> Mux/4
  Compare To Constant2/1 -> Mux/3
  Compare To Constant1/1 -> Mux/2
  Compare To Constant/1 -> Mux/1
  Mux/1 -> Out1/1
  In1/1 -> Compare To Constant4/1, Compare To Constant5/1, Compare To Constant6/1, Compare To Constant7/1, Compare To Constant3/1, Compare To Constant2/1, Compare To Constant1/1, Compare To Constant/1

== system BEML_EMU_DoorsInput_Lib/DoorsInterface/DoorsInputAdapter/VehicleInputAdapter/DoorsInputs/Subsystem/Subsystem9 ==
  In1 : Inport
  Compare To Constant : simulink/Logic and Bit Operations/Compare To Constant  relop===  const=1  OutDataTypeStr=boolean
  Compare To Constant1 : simulink/Logic and Bit Operations/Compare To Constant  relop===  const=2  OutDataTypeStr=boolean
  Compare To Constant2 : simulink/Logic and Bit Operations/Compare To Constant  relop===  const=3  OutDataTypeStr=boolean
  Compare To Constant3 : simulink/Logic and Bit Operations/Compare To Constant  relop===  const=4  OutDataTypeStr=boolean
  Compare To Constant4 : simulink/Logic and Bit Operations/Compare To Constant  relop===  const=5  OutDataTypeStr=boolean
  Compare To Constant5 : simulink/Logic and Bit Operations/Compare To Constant  relop===  const=6  OutDataTypeStr=boolean
  Compare To Constant6 : simulink/Logic and Bit Operations/Compare To Constant  relop===  const=7  OutDataTypeStr=boolean
  Compare To Constant7 : simulink/Logic and Bit Operations/Compare To Constant  relop===  const=8  OutDataTypeStr=boolean
  Mux : Mux  Inputs=8
  Out1 : Outport
  wires:
  In1/1 -> Compare To Constant/1, Compare To Constant1/1, Compare To Constant2/1, Compare To Constant3/1, Compare To Constant7/1, Compare To Constant6/1, Compare To Constant5/1, Compare To Constant4/1
  Mux/1 -> Out1/1
  Compare To Constant/1 -> Mux/1
  Compare To Constant1/1 -> Mux/2
  Compare To Constant2/1 -> Mux/3
  Compare To Constant3/1 -> Mux/4
  Compare To Constant4/1 -> Mux/5
  Compare To Constant5/1 -> Mux/6
  Compare To Constant6/1 -> Mux/7
  Compare To Constant7/1 -> Mux/8

== system BEML_EMU_DoorsInput_Lib/DoorsInterface/DoorsInputAdapter/VehicleInputAdapter/DoorsInputs/DoorsArrangement/Subsystem1/For Each Subsystem2 ==
  Source1 : Inport  Partition=on  PartitionDimension=1  PartitionWidth=1  PartitionOffset=0
  Source2 : Inport  Port=2  Partition=on  PartitionDimension=1  PartitionWidth=1  PartitionOffset=0
  Orientation : Inport  Port=3
  For Each : ForEach  DisableCoverage=on
  Orientation Swap : VectorOperationsLib/Orientation Swap
      settings: SourceProductName=Sydac Utilities
  WireState1 : Outport  ConcatenationDimension=1
  WireState2 : Outport  Port=2  ConcatenationDimension=1
  wires:
  Source1/1 -> Orientation Swap/1
  Orientation Swap/1 -> WireState1/1
  Orientation Swap/2 -> WireState2/1
  Source2/1 -> Orientation Swap/2
  Orientation/1 -> Orientation Swap/3
